simulink model "pid_test"  (R2016a)
settings: Solver=VariableStepAuto  StartTime=0.0  StopTime=50.0  RelTol=1e-3
undefined symbols (not defined in the file): KD, KI, Kp
settings Model: Creator=shohei  LastModifiedBy=shohei

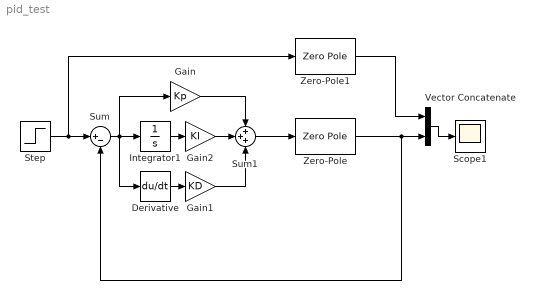
== system pid_test ==
  Derivative : Derivative
  Gain : Gain  Gain=Kp
  Gain1 : Gain  Gain=KD
  Gain2 : Gain  Gain=KI
  Integrator1 : Integrator
  Scope1 : Scope
  Step : Step  SampleTime=0
  Sum : Sum  Inputs=|+-
  Sum1 : Sum  Inputs=+++
  Vector Concatenate : Concatenate
  Zero-Pole : ZeroPole  Poles=[0 -1]  Gain=[2]
  Zero-Pole1 : ZeroPole  Poles=[0 -1]  Gain=[2]
  wires:
  Zero-Pole/1 -> Vector Concatenate/2, Sum/2
  Integrator1/1 -> Gain2/1
  Derivative/1 -> Gain1/1
  Sum/1 -> Gain/1, Derivative/1, Integrator1/1
  Step/1 -> Zero-Pole1/1, Sum/1
  Gain2/1 -> Sum1/2
  Gain/1 -> Sum1/1
  Gain1/1 -> Sum1/3
  Sum1/1 -> Zero-Pole/1
  Vector Concatenate/1 -> Scope1/1
  Zero-Pole1/1 -> Vector Concatenate/1
